simulink model "ModelPendulumTest"  (R2024a)
settings: Solver=VariableStepAuto  StartTime=0.0  StopTime=60  RelTol=1e-3
undefined symbols (not defined in the file): control, den_mf_track, DiscIntNeverNeededParam, K_controller, K_controller2, model, num_mf_track, R, r0_meq, r1_meq, r2_meq, s1_meq, T, Ts
libraries: simulink x1
settings Model: Creator=Douglas  LastModifiedBy=Douglas

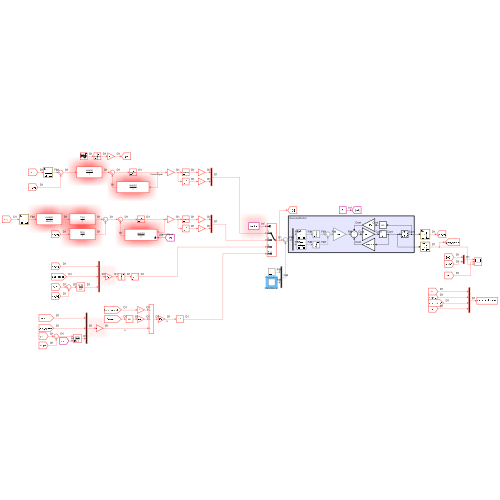
[thumbnail: Simulink's stored preview of the top-level diagram]
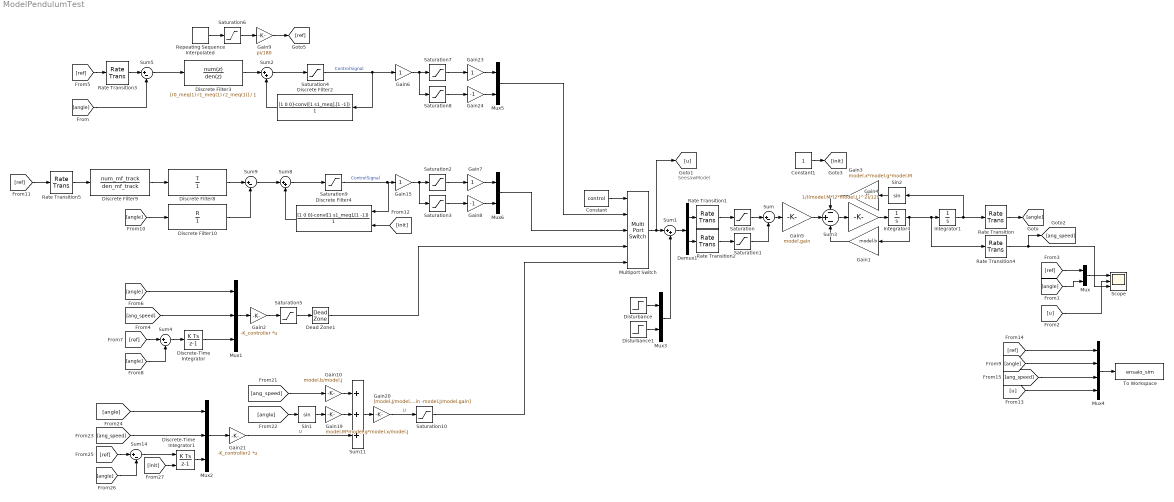
== system ModelPendulumTest ==
  note: SeesawModel
  Constant : Constant  Value=control
  Constant1 : Constant
  Dead Zone1 : DeadZone  LowerValue=-0  UpperValue=0
  Demux1 : Demux  Outputs=2
  Discrete Filter10 : DiscreteFilter  Numerator=R  Denominator=1
  Discrete Filter2 : DiscreteFilter  Numerator=[1 0 0]-conv([1 s1_meq],[1 -1])  Denominator=1
  Discrete Filter3 : DiscreteFilter  Numerator=[r0_meq(1) r1_meq(1) r2_meq(1)]  Denominator=1
  Discrete Filter4 : DiscreteFilter  Numerator=[1 0 0]-conv([1 s1_meq],[1 -1])  Denominator=1  ExternalReset=Rising
      settings: InputPortMap=u0,r7
  Discrete Filter8 : DiscreteFilter  Numerator=T  Denominator=1
  Discrete Filter9 : DiscreteFilter  Numerator=num_mf_track  Denominator=den_mf_track
  Discrete-Time Integrator : DiscreteIntegrator  SampleTime=-1  ICPrevOutput=DiscIntNeverNeededParam  ICPrevScaledInput=DiscIntNeverNeededParam
  Discrete-Time Integrator1 : DiscreteIntegrator  ExternalReset=rising  SampleTime=-1  ICPrevOutput=DiscIntNeverNeededParam  ICPrevScaledInput=DiscIntNeverNeededParam
  Disturbance : Step  Time=5+15  After=0.04  SampleTime=0
  Disturbance1 : Step  Time=20+15  After=0.04  SampleTime=0
  Gain1 : Gain  Gain=model.b
  Gain10 : Gain  Gain=model.b/model.J
  Gain{6..7,15,23} (4 alike) : Gain
  Gain19 : Gain  Gain=model.M*model.g*model.x/model.J
  Gain2 : Gain  Gain=-K_controller  Multiplication=Matrix(K*u)
  Gain20 : Gain  Gain=[model.J/model.gain -model.J/model.gain]
  Gain21 : Gain  Gain=-K_controller2  Multiplication=Matrix(K*u)
  Gain24 : Gain  Gain=-1
  Gain3 : Gain  Gain=model.x*model.g*model.M
  Gain4 : Gain  Gain=1/((model.M*(2*model.L)^2)/12)
  Gain5 : Gain  Gain=model.gain
  Gain8 : Gain  Gain=-1
  Gain9 : Gain  Gain=pi/180
  Integrator1 : Integrator  WrapState=on
  Integrator4 : Integrator
  Multiport Switch : MultiPortSwitch  Inputs=4  SaturateOnIntegerOverflow=off  InputSameDT=off
  Mux{,3,5..6} (4 alike) : Mux  Inputs=2
  Mux1 : Mux  Inputs=3
  Mux2 : Mux  Inputs=3
  Mux4 : Mux
  Rate Transition : RateTransition  OutPortSampleTime=Ts
  Rate Transition{1..3,5} (4 alike) : RateTransition
  Rate Transition4 : RateTransition  OutPortSampleTime=Ts
  Repeating Sequence Interpolated : simulink/Sources/Repeating Sequence Interpolated  OutValues=[0 0 20 20 -45 -45 60 60].'  TimeValues=[0 15 15+Ts 30 30+Ts 45 45+Ts 60].'  LookUpMeth=Interpolation-Use End Values  tsamp=Ts  OutMin=[]  OutMax=[]  OutDataTypeStr=double  OutputDataTypeScalingMode=double  OutDataType=fixdt(0,8)  OutScaling=2^-10
  Saturation{,1..2,5,7,10} (6 alike) : Saturate  UpperLimit=1  LowerLimit=0
  Saturation3 : Saturate  UpperLimit=0  LowerLimit=-1
  Saturation4 : Saturate  UpperLimit=1  LowerLimit=-1
  Saturation6 : Saturate  UpperLimit=140  LowerLimit=-140
  Saturation8 : Saturate  UpperLimit=0  LowerLimit=-1
  Saturation9 : Saturate  UpperLimit=1  LowerLimit=-1
  Scope : Scope  NumInputPorts=3
  Sin1 : Trigonometry
  Sin2 : Trigonometry
  Sum : Sum  Inputs=|+-  OutDataTypeStr=double
  Sum1 : Sum  Inputs=|++
  Sum11 : Sum  Inputs=+++
  Sum14 : Sum  Inputs=|+-
  Sum2 : Sum  Inputs=|++
  Sum3 : Sum  Inputs=-+-
  Sum4 : Sum  Inputs=|+-
  Sum5 : Sum  Inputs=|+-
  Sum8 : Sum  Inputs=|++  OutDataTypeStr=single
  Sum9 : Sum  Inputs=|+-  OutDataTypeStr=Inherit: Inherit via back propagation
  To Workspace : ToWorkspace  VariableName=ensaio_sim  SaveFormat=Structure With Time  SampleTime=Ts
  wires:
  Integrator1/1 -> Rate Transition/1, Sin2/1
  Saturation1/1 -> Sum/2
  Saturation/1 -> Sum/1
  Rate Transition2/1 -> Saturation1/1
  Sum/1 -> Gain5/1
  Rate Transition1/1 -> Saturation/1
  Gain4/1 -> Integrator4/1
  Gain3/1 -> Sum3/1
  Gain5/1 -> Sum3/2
  Sum3/1 -> Gain4/1
  Sin2/1 -> Gain3/1
  Gain1/1 -> Sum3/3
  Integrator4/1 -> Rate Transition4/1, Integrator1/1, Gain1/1
  Sum5/1 -> Discrete Filter3/1
  Discrete Filter3/1 -> Sum2/1
  Saturation4/1 -> Gain6/1, Discrete Filter2/1  "ControlSignal"
  Rate Transition/1 -> [angle]
  [angle] -> Sum5/2
  [angle] -> Mux/2
  [u] -> Scope/2
  [ref] -> Mux/1
  Mux/1 -> Scope/1
  Discrete Filter2/1 -> Sum2/2
  Sum2/1 -> Saturation4/1
  Rate Transition3/1 -> Sum5/1
  Gain6/1 -> Saturation8/1, Saturation7/1
  [ref] -> Rate Transition3/1
  [init] -> Discrete Filter4/2
  Saturation6/1 -> Gain9/1
  Discrete Filter9/1 -> Discrete Filter8/1
  Rate Transition5/1 -> Discrete Filter9/1
  Sum8/1 -> Saturation9/1
  [ref] -> Rate Transition5/1
  Discrete Filter10/1 -> Sum9/2
  [angle] -> Discrete Filter10/1
  Discrete Filter4/1 -> Sum8/2
  Saturation9/1 -> Discrete Filter4/1, Gain15/1  "ControlSignal"
  Sum9/1 -> Sum8/1
  Discrete Filter8/1 -> Sum9/1
  Gain9/1 -> [ref]
  Repeating Sequence Interpolated/1 -> Saturation6/1
  Rate Transition4/1 -> Scope/3, [ang_speed]
  [ref] -> Sum4/1
  [angle] -> Sum4/2
  Sum4/1 -> Discrete-Time Integrator/1
  [angle] -> Mux1/1
  [ang_speed] -> Mux1/2
  Discrete-Time Integrator/1 -> Mux1/3
  Mux1/1 -> Gain2/1
  Gain2/1 -> Saturation5/1
  Saturation5/1 -> Dead Zone1/1
  Dead Zone1/1 -> Multiport Switch/4
  Saturation8/1 -> Gain24/1
  [angle] -> Sin1/1
  Gain10/1 -> Sum11/1
  Sum11/1 -> Gain20/1
  Sin1/1 -> Gain19/1
  [ang_speed] -> Gain10/1
  Discrete-Time Integrator1/1 -> Mux2/3
  Gain19/1 -> Sum11/2
  Sum14/1 -> Discrete-Time Integrator1/1
  [ref] -> Sum14/1
  Mux2/1 -> Gain21/1
  [ang_speed] -> Mux2/2
  Saturation7/1 -> Gain23/1
  [angle] -> Mux2/1
  [angle] -> Sum14/2
  [init] -> Discrete-Time Integrator1/2
  Constant1/1 -> [init]
  Gain23/1 -> Mux5/1
  Gain24/1 -> Mux5/2
  Gain8/1 -> Mux6/2
  Gain7/1 -> Mux6/1
  Saturation2/1 -> Gain7/1
  Saturation3/1 -> Gain8/1
  Gain15/1 -> Saturation2/1, Saturation3/1
  Demux1/1 -> Rate Transition1/1
  Demux1/2 -> Rate Transition2/1
  Multiport Switch/1 -> [u], Sum1/1
  Mux5/1 -> Multiport Switch/2
  Mux6/1 -> Multiport Switch/3
  Gain20/1 -> Saturation10/1  "U"
  Constant/1 -> Multiport Switch/1
  Gain21/1 -> Sum11/3  "U"
  Saturation10/1 -> Multiport Switch/5
  Sum1/1 -> Demux1/1
  Disturbance/1 -> Mux3/1
  Disturbance1/1 -> Mux3/2
  Mux3/1 -> Sum1/2
  [ref] -> Mux4/1
  [angle] -> Mux4/2
  [ang_speed] -> Mux4/3
  [u] -> Mux4/4
  Mux4/1 -> To Workspace/1
